simulink model "roverClosed_states_hw"  (R2024a)
settings: Solver=FixedStepAuto  StartTime=0.0  StopTime=100  FixedStep=TS  RelTol=1e-3  EnableMultiTasking=on
PostLoadFcn:
  | params
  | load('motorResponse.mat')
model workspace (MAT data in the model file):
  TS = 0.01
undefined symbols (not defined in the file): L, PWMcmdMono, r, speedMono, StartTheta
libraries: arduinomotorcarrierlib x4, simulink_extras x4, slpidlib x2
settings Model: ExtModeTrigDuration=2  Creator=jmodiset  LastModifiedBy=Sheen
settings SolverCC: AlgebraicLoopSolver=TrustRegion
settings DataIOCC: ReturnWorkspaceOutputs=off
settings OptimizationCC: PassReuseOutputArgsThreshold=0  MaxStackSize=64
settings DebuggingCC: UnderspecifiedInitializationDetection=Classic  MergeDetectMultiDrivingBlocksExec=none  ParameterTunabilityLossMsg=error  UnconnectedInputMsg=warning  UnconnectedOutputMsg=warning  UnconnectedLineMsg=warning  PregeneratedLibrarySubsystemCodeDiagnostic=none  ArithmeticOperatorsInVariantConditions=warning
settings HardwareCC: ProdBitPerPointer=32  ProdBitPerSizeT=32  ProdBitPerPtrDiffT=32  ProdLargestAtomicInteger=Long  ProdLargestAtomicFloat=Double  ProdWordSize=32  ProdHWDeviceType=ARM Compatible->ARM Cortex  UseEmbeddedCoderFeatures=off  UseSimulinkCoderFeatures=off
settings ModelReferenceCC: EnableRefExpFcnMdlSchedulingChecks=on
settings SFSimCC: SimUseLocalCustomCode=off  MATLABDynamicMemAlloc=off  CustomCodeUndefinedFunction=UseInterfaceOnly
settings RTWCC: Description=Embedded Coder  SystemTargetFile=ert.tlc  HardwareBoard=Arduino Nano 33 IoT  TemplateMakefile=ert_default_tmf  RTWUseLocalCustomCode=off  Toolchain=Arduino ARM  BuildConfiguration=Faster Runs  GPUComputeCapability=3.5
settings CodeAppCC: ForceParamTrailComments=on  OperatorAnnotations=on
settings ERTTargetCC: ERTCustomFileBanners=off  SupportContinuousTime=on  SupportNonInlinedSFcns=on  RemoveResetFunc=off  SupportVariableSizeSignals=on  ModelStepFunctionPrototypeControlCompliant=off  ExtModeStaticAllocSize=8192

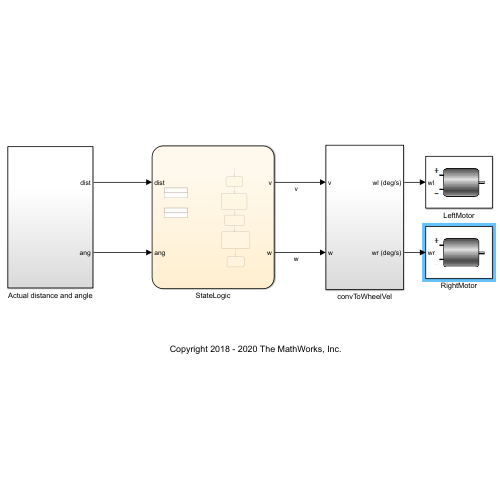
[thumbnail: Simulink's stored preview of the top-level diagram]
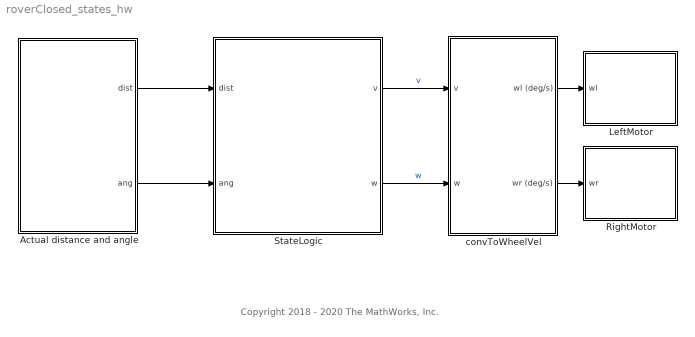
== system roverClosed_states_hw ==
  note: Copyright 2018 - 2020 The MathWorks, Inc.
  Actual distance and angle : Subsystem
  LeftMotor : Subsystem
      mask Display:
      | color('white');
      | plot([100,100,100,100]*1,[100,100,100,100]*1);
      | plot([100,100,100,100]*0,[100,100,100,100]*0);
      | sppkgroot = strrep(codertarget.arduinobase.internal.getBaseSpPkgRootDir(),'\','/');
      | image(fullfile(sppkgroot,'resources','dcmotor.png'),'center')
  RightMotor : Subsystem
      mask Display:
      | color('white');
      | plot([100,100,100,100]*1,[100,100,100,100]*1);
      | plot([100,100,100,100]*0,[100,100,100,100]*0);
      | sppkgroot = strrep(codertarget.arduinobase.internal.getBaseSpPkgRootDir(),'\','/');
      | image(fullfile(sppkgroot,'resources','dcmotor.png'),'center')
  StateLogic : Stateflow chart  TreatAsAtomicUnit=on
  convToWheelVel : Subsystem
  wires:
  Actual distance and angle/1(dist) -> StateLogic/1(dist)
  Actual distance and angle/2(ang) -> StateLogic/2(ang)
  convToWheelVel/1(wl (deg/s)) -> LeftMotor/1(wl)
  StateLogic/1(v) -> convToWheelVel/1(v)  "v"
  convToWheelVel/2(wr (deg/s)) -> RightMotor/1(wr)
  StateLogic/2(w) -> convToWheelVel/2(w)  "w"

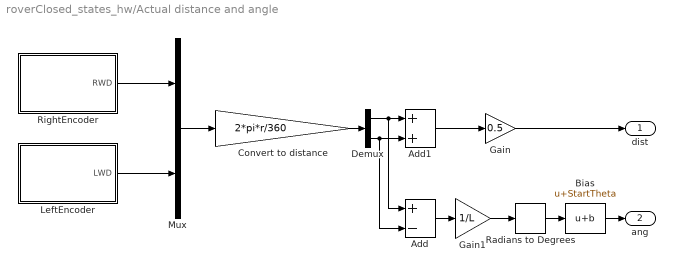
== system roverClosed_states_hw/Actual distance and angle ==
  Add : Sum  Inputs=+-
  Add1 : Sum
  Bias : Bias  Bias=StartTheta  SaturateOnIntegerOverflow=off
  Convert to distance : Gain  Gain=2*pi*r/360
  Demux : Demux  Outputs=2
  Gain : Gain  Gain=0.5
  Gain1 : Gain  Gain=1/L
  LeftEncoder : Subsystem
  Mux : Mux  Inputs=2
  Radians to Degrees : simulink_extras/Transformations/Radians to Degrees
  RightEncoder : Subsystem
  dist : Outport  VectorParamsAs1DForOutWhenUnconnected=off
  ang : Outport  Port=2  VectorParamsAs1DForOutWhenUnconnected=off
  wires:
  RightEncoder/1(RWD) -> Mux/1
  Gain1/1 -> Radians to Degrees/1
  Add/1 -> Gain1/1
  Demux/2 -> Add1/2, Add/2
  Convert to distance/1 -> Demux/1
  Demux/1 -> Add1/1, Add/1
  Mux/1 -> Convert to distance/1
  LeftEncoder/1(LWD) -> Mux/2
  Radians to Degrees/1 -> Bias/1
  Add1/1 -> Gain/1
  Gain/1 -> dist/1
  Bias/1 -> ang/1

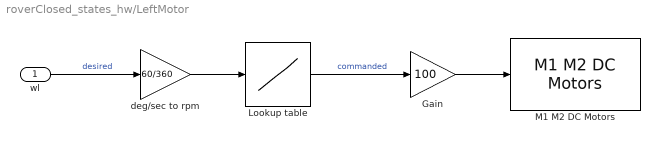
== system roverClosed_states_hw/LeftMotor ==
  wl : Inport
  Gain : Gain  Gain=100
  Lookup table : Lookup_n-D  NumberOfTableDimensions=1  BreakpointsForDimension1=speedMono  Table=PWMcmdMono  UseLastTableValue=on  InternalRulePriority=Speed  RndMeth=Simplest
  M1 M2 DC Motors : arduinomotorcarrierlib/M1 M2 DC Motors  SlaveAddress=uint8( hex2dec( '66' ) )  blockPlatform=ARDUINO  MotorNumber=M2  MotorCarrierPWMFreq=100
  deg/sec to rpm : Gain  Gain=60/360
  wires:
  wl/1 -> deg/sec to rpm/1  "desired"
  Lookup table/1 -> Gain/1  "commanded"
  deg/sec to rpm/1 -> Lookup table/1
  Gain/1 -> M1 M2 DC Motors/1

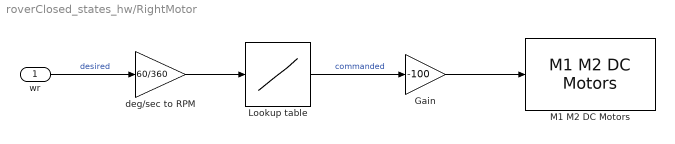
== system roverClosed_states_hw/RightMotor ==
  wr : Inport
  Gain : Gain  Gain=-100
  Lookup table : Lookup_n-D  NumberOfTableDimensions=1  BreakpointsForDimension1=speedMono  Table=PWMcmdMono  UseLastTableValue=on  InternalRulePriority=Speed  RndMeth=Simplest
  M1 M2 DC Motors : arduinomotorcarrierlib/M1 M2 DC Motors  SlaveAddress=uint8( hex2dec( '66' ) )  blockPlatform=ARDUINO  MotorNumber=M1  MotorCarrierPWMFreq=100
  deg/sec to RPM : Gain  Gain=60/360
  wires:
  wr/1 -> deg/sec to RPM/1  "desired"
  Lookup table/1 -> Gain/1  "commanded"
  Gain/1 -> M1 M2 DC Motors/1
  deg/sec to RPM/1 -> Lookup table/1

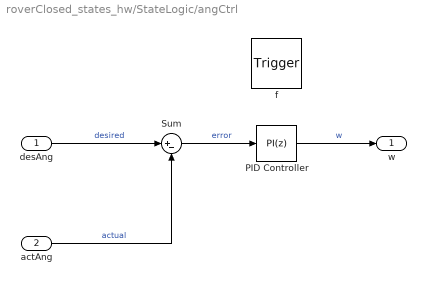
== system roverClosed_states_hw/StateLogic/angCtrl ==
  desAng : Inport  OutDataTypeStr=double  PortDimensions=1
  actAng : Inport  Port=2  OutDataTypeStr=double  PortDimensions=1
  f : TriggerPort  TriggerType=function-call  VariantControl=(inherit)
      settings: CopyFcn=Stateflow.SLINSF.SimulinkMan.removeBlockPreDeleteFcn  PreDeleteFcn=Stateflow.SLINSF.SimulinkMan.unsafePredeleteFcn
  PID Controller : slpidlib/PID Controller  Controller=PI  Form=Parallel  TimeDomain=Discrete-time  UseExternalTs=off  SampleTime=-1  IntegratorMethod=Forward Euler  FilterMethod=Forward Euler  ControllerParametersSource=internal  P=2  I=0.2  UseKiTs=off  D=0  UseExternalDerivativeSource=off  N=100  UseFilter=on  TunerSelectOption=Transfer Function Based (PID Tuner App)  InitialConditionSource=internal  InitialConditionForIntegrator=0  InitialConditionForFilter=0  DifferentiatorICPrevScaledInput=0  ExternalReset=none  TrackingMode=off  Kt=1  LimitOutput=off  SatLimitsSource=internal  UpperSaturationLimit=inf  LowerSaturationLimit=-inf  LinearizeAsGain=on  AntiWindupMode=none  Kb=1  LimitIntegrator=off  UpperIntegratorSaturationLimit=inf  LowerIntegratorSaturationLimit=-inf  POutMin=[]  POutMax=[]  IOutMin=[]  IOutMax=[]  DOutMin=[]  DOutMax=[]  NOutMin=[]  NOutMax=[]  SumOutMin=[]  SumOutMax=[]  SaturationOutMin=[]  SaturationOutMax=[]  PParamMin=[]  PParamMax=[]  IParamMin=[]  IParamMax=[]  DParamMin=[]  DParamMax=[]  NParamMin=[]  NParamMax=[]  KbParamMin=[]  KbParamMax=[]  KtParamMin=[]  KtParamMax=[]  KbOutMin=[]  KbOutMax=[]  KtOutMin=[]  KtOutMax=[]  IntegratorOutMin=[]  IntegratorOutMax=[]  FilterOutMin=[]  FilterOutMax=[]  SumI1OutMin=[]  SumI1OutMax=[]  SumI2OutMin=[]  SumI2OutMax=[]  SumI3OutMin=[]  SumI3OutMax=[]  SumI4OutMin=[]  SumI4OutMax=[]  SumDOutMin=[]  SumDOutMax=[]  DifferentiatorOutMin=[]  DifferentiatorOutMax=[]  FilterDiffOutCoefMin=[]  FilterDiffOutCoefMax=[]  ReciprocalOutMin=[]  ReciprocalOutMax=[]  SumDenOutMin=[]  SumDenOutMax=[]  SumNumOutMin=[]  SumNumOutMax=[]  DivideOutMin=[]  DivideOutMax=[]  UdiffTsProdOutMin=[]  UdiffTsProdOutMax=[]  NTsProdOutMin=[]  NTsProdOutMax=[]  UintegralTsProdOutMin=[]  UintegralTsProdOutMax=[]  UngainTsProdOutMin=[]  UngainTsProdOutMax=[]  ClampingZeroOutDataTypeStr=Inherit: Inherit via back propagation  ClampingZeroOutMin=[]  ClampingZeroOutMax=[]  FilterDenConstantOutDataTypeStr=Inherit: Inherit via back propagation  FilterDenConstantOutMin=[]  FilterDenConstantOutMax=[]  PCopyOutDataTypeStr=Inherit: Inherit via back propagation  PCopyOutMin=[]  PCopyOutMax=[]  NCopyOutDataTypeStr=Inherit: Inherit via back propagation  NCopyOutMin=[]  NCopyOutMax=[]  IntegratorContinuousStateAttributes=''  IntegratorStateMustResolveToSignalObject=off  IntegratorRTWStateStorageClass=Auto  FilterContinuousStateAttributes=''  FilterStateMustResolveToSignalObject=off  FilterRTWStateStorageClass=Auto  ParallelPVariant=InternalParameters  IdealPVariant=Disabled  IVariant=InternalParameters  DVariant=Disabled  IntegratorVariant=Discrete  SatVariant=Disabled  AWVariant=Passthrough  PCopyVariant=Disabled  TRVariant=Disabled  FdbkBlocksVariant=Forward  IdealPFdbkVariant=Disabled  SatFdbkVariant=Disabled  DerivativeFilterVariant=Disabled  NVariant=Disabled  NCopyVariant=Disabled_SignalSpec  FilterICVariant=Disabled  IntegratorICVariant=InternalICs  ExternalResetVariant=Disabled  TRSumVariant=Passthrough  SumFdbkVariant=Disabled  SumVariant=Sum_PI  TsampFilterVariant=InternalTs  TsampNgainVariant=Passthrough  TsampIntegralVariant=Disabled_SignalSpec  ExternalSaturationOutDataTypeStr=Inherit: Same as second input  DerivativeSourceVariant=Disabled
  Sum : Sum  Inputs=|+-
  w : Outport  VectorParamsAs1DForOutWhenUnconnected=off
  wires:
  actAng/1 -> Sum/2  "actual"
  desAng/1 -> Sum/1  "desired"
  PID Controller/1 -> w/1  "w"
  Sum/1 -> PID Controller/1  "error"

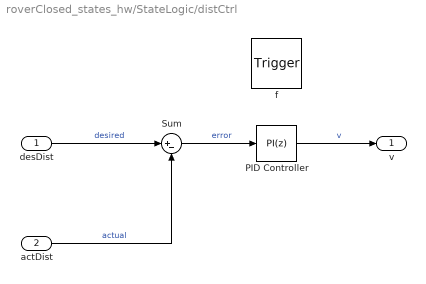
== system roverClosed_states_hw/StateLogic/distCtrl ==
  desDist : Inport  OutDataTypeStr=double  PortDimensions=1
  actDist : Inport  Port=2  OutDataTypeStr=double  PortDimensions=1
  f : TriggerPort  TriggerType=function-call  VariantControl=(inherit)
      settings: CopyFcn=Stateflow.SLINSF.SimulinkMan.removeBlockPreDeleteFcn  PreDeleteFcn=Stateflow.SLINSF.SimulinkMan.unsafePredeleteFcn
  PID Controller : slpidlib/PID Controller  Controller=PI  Form=Parallel  TimeDomain=Discrete-time  UseExternalTs=off  SampleTime=-1  IntegratorMethod=Forward Euler  FilterMethod=Forward Euler  ControllerParametersSource=internal  P=0.2  I=0.001  UseKiTs=off  D=0  UseExternalDerivativeSource=off  N=100  UseFilter=on  TunerSelectOption=Transfer Function Based (PID Tuner App)  InitialConditionSource=internal  InitialConditionForIntegrator=0  InitialConditionForFilter=0  DifferentiatorICPrevScaledInput=0  ExternalReset=none  TrackingMode=off  Kt=1  LimitOutput=off  SatLimitsSource=internal  UpperSaturationLimit=inf  LowerSaturationLimit=-inf  LinearizeAsGain=on  AntiWindupMode=none  Kb=1  LimitIntegrator=off  UpperIntegratorSaturationLimit=inf  LowerIntegratorSaturationLimit=-inf  POutMin=[]  POutMax=[]  IOutMin=[]  IOutMax=[]  DOutMin=[]  DOutMax=[]  NOutMin=[]  NOutMax=[]  SumOutMin=[]  SumOutMax=[]  SaturationOutMin=[]  SaturationOutMax=[]  PParamMin=[]  PParamMax=[]  IParamMin=[]  IParamMax=[]  DParamMin=[]  DParamMax=[]  NParamMin=[]  NParamMax=[]  KbParamMin=[]  KbParamMax=[]  KtParamMin=[]  KtParamMax=[]  KbOutMin=[]  KbOutMax=[]  KtOutMin=[]  KtOutMax=[]  IntegratorOutMin=[]  IntegratorOutMax=[]  FilterOutMin=[]  FilterOutMax=[]  SumI1OutMin=[]  SumI1OutMax=[]  SumI2OutMin=[]  SumI2OutMax=[]  SumI3OutMin=[]  SumI3OutMax=[]  SumI4OutMin=[]  SumI4OutMax=[]  SumDOutMin=[]  SumDOutMax=[]  DifferentiatorOutMin=[]  DifferentiatorOutMax=[]  FilterDiffOutCoefMin=[]  FilterDiffOutCoefMax=[]  ReciprocalOutMin=[]  ReciprocalOutMax=[]  SumDenOutMin=[]  SumDenOutMax=[]  SumNumOutMin=[]  SumNumOutMax=[]  DivideOutMin=[]  DivideOutMax=[]  UdiffTsProdOutMin=[]  UdiffTsProdOutMax=[]  NTsProdOutMin=[]  NTsProdOutMax=[]  UintegralTsProdOutMin=[]  UintegralTsProdOutMax=[]  UngainTsProdOutMin=[]  UngainTsProdOutMax=[]  ClampingZeroOutDataTypeStr=Inherit: Inherit via back propagation  ClampingZeroOutMin=[]  ClampingZeroOutMax=[]  FilterDenConstantOutDataTypeStr=Inherit: Inherit via back propagation  FilterDenConstantOutMin=[]  FilterDenConstantOutMax=[]  PCopyOutDataTypeStr=Inherit: Inherit via back propagation  PCopyOutMin=[]  PCopyOutMax=[]  NCopyOutDataTypeStr=Inherit: Inherit via back propagation  NCopyOutMin=[]  NCopyOutMax=[]  IntegratorContinuousStateAttributes=''  IntegratorStateMustResolveToSignalObject=off  IntegratorRTWStateStorageClass=Auto  FilterContinuousStateAttributes=''  FilterStateMustResolveToSignalObject=off  FilterRTWStateStorageClass=Auto  ParallelPVariant=InternalParameters  IdealPVariant=Disabled  IVariant=InternalParameters  DVariant=Disabled  IntegratorVariant=Discrete  SatVariant=Disabled  AWVariant=Passthrough  PCopyVariant=Disabled  TRVariant=Disabled  FdbkBlocksVariant=Forward  IdealPFdbkVariant=Disabled  SatFdbkVariant=Disabled  DerivativeFilterVariant=Disabled  NVariant=Disabled  NCopyVariant=Disabled_SignalSpec  FilterICVariant=Disabled  IntegratorICVariant=InternalICs  ExternalResetVariant=Disabled  TRSumVariant=Passthrough  SumFdbkVariant=Disabled  SumVariant=Sum_PI  TsampFilterVariant=InternalTs  TsampNgainVariant=Passthrough  TsampIntegralVariant=Disabled_SignalSpec  ExternalSaturationOutDataTypeStr=Inherit: Same as second input  DerivativeSourceVariant=Disabled
  Sum : Sum  Inputs=|+-
  v : Outport  VectorParamsAs1DForOutWhenUnconnected=off
  wires:
  actDist/1 -> Sum/2  "actual"
  desDist/1 -> Sum/1  "desired"
  PID Controller/1 -> v/1  "v"
  Sum/1 -> PID Controller/1  "error"

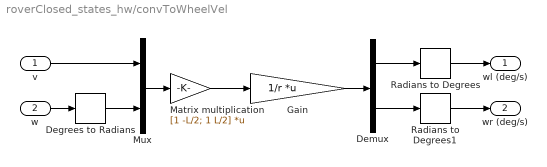
== system roverClosed_states_hw/convToWheelVel ==
  v : Inport
  w : Inport  Port=2
  " Gain" : Gain  Gain=1/r  Multiplication=Matrix(K*u)
  Degrees to Radians : simulink_extras/Transformations/Degrees to Radians
  Demux : Demux  Outputs=2
  Matrix multiplication : Gain  Gain=[1 -L/2; 1 L/2]  Multiplication=Matrix(K*u)
  Mux : Mux  Inputs=2
  Radians to Degrees : simulink_extras/Transformations/Radians to Degrees
  Radians to Degrees1 : simulink_extras/Transformations/Radians to Degrees
  wl (deg/s) : Outport  VectorParamsAs1DForOutWhenUnconnected=off
  wr (deg/s) : Outport  Port=2  VectorParamsAs1DForOutWhenUnconnected=off
  wires:
  " Gain"/1 -> Demux/1
  Matrix multiplication/1 -> " Gain"/1
  v/1 -> Mux/1
  Mux/1 -> Matrix multiplication/1
  Demux/1 -> Radians to Degrees/1
  Demux/2 -> Radians to Degrees1/1
  w/1 -> Degrees to Radians/1
  Radians to Degrees/1 -> wl (deg/s)/1
  Radians to Degrees1/1 -> wr (deg/s)/1
  Degrees to Radians/1 -> Mux/2

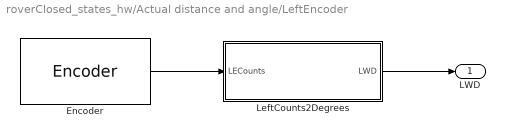
== system roverClosed_states_hw/Actual distance and angle/LeftEncoder ==
  Encoder : arduinomotorcarrierlib/Encoder  SlaveAddress=uint8( hex2dec( '66' ) )  blockPlatform=ARDUINO  Encoder=2  ShowSpeed=off  ResetOption=on  SampleTime=0.01
  LeftCounts2Degrees : Subsystem
  LWD : Outport  VectorParamsAs1DForOutWhenUnconnected=off
  wires:
  LeftCounts2Degrees/1(LWD) -> LWD/1
  Encoder/1 -> LeftCounts2Degrees/1(LECounts)

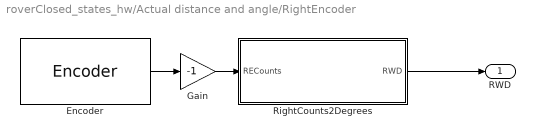
== system roverClosed_states_hw/Actual distance and angle/RightEncoder ==
  Encoder : arduinomotorcarrierlib/Encoder  SlaveAddress=uint8( hex2dec( '66' ) )  blockPlatform=ARDUINO  Encoder=1  ShowSpeed=off  ResetOption=on  SampleTime=0.01
  Gain : Gain  Gain=-1
  RightCounts2Degrees : Subsystem
  RWD : Outport  VectorParamsAs1DForOutWhenUnconnected=off
  wires:
  RightCounts2Degrees/1(RWD) -> RWD/1
  Encoder/1 -> Gain/1
  Gain/1 -> RightCounts2Degrees/1(RECounts)

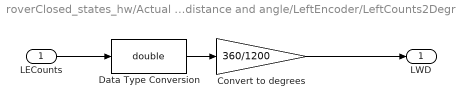
== system roverClosed_states_hw/Actual distance and angle/LeftEncoder/LeftCounts2Degrees ==
  LECounts : Inport
  Convert to degrees : Gain  Gain=360/1200
  Data Type Conversion : DataTypeConversion  OutDataTypeStr=double  SaturateOnIntegerOverflow=off  RndMeth=Floor
  LWD : Outport  VectorParamsAs1DForOutWhenUnconnected=off
  wires:
  LECounts/1 -> Data Type Conversion/1
  Data Type Conversion/1 -> Convert to degrees/1
  Convert to degrees/1 -> LWD/1

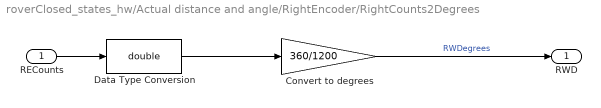
== system roverClosed_states_hw/Actual distance and angle/RightEncoder/RightCounts2Degrees ==
  RECounts : Inport
  Convert to degrees : Gain  Gain=360/1200
  Data Type Conversion : DataTypeConversion  OutDataTypeStr=double  SaturateOnIntegerOverflow=off  RndMeth=Floor
  RWD : Outport  VectorParamsAs1DForOutWhenUnconnected=off
  wires:
  Data Type Conversion/1 -> Convert to degrees/1
  RECounts/1 -> Data Type Conversion/1
  Convert to degrees/1 -> RWD/1  "RWDegrees"

== stateflow chart roverClosed_states_hw/StateLogic ==
  state StopFirst
    entry:
    v = 0; w= 0;
  state v = distCtrl(desDist,actDist) [function]
  state MoveForward
    entry:
    desDist = 30;
    during, exit:
    v = distCtrl(desDist,dist);
    w = 0;
  state w = angCtrl(desAng,actAng) [function]
  state Pause
    entry:
    v = 0;
    w = 0;
  state Turn
    entry:
    desAng = 180;
    during, exit:
    v = 0;
    w = angCtrl(desAng,ang);
  state Stop
    entry:
    v = 0;
    w = 0;
  (default) -> StopFirst
  StopFirst -> MoveForward : after(1,sec)
  MoveForward -> Pause : [abs(desDist - dist) < 0.5]
  Pause -> Turn : after(1,sec)
  Turn -> Stop : [abs(desAng - ang) < 2]
  data: desDist function_input double size=1; actDist function_input double size=1; v function_output; desAng function_input double size=1; actAng function_input double size=1; w function_output; dist input; ang input; v output; w output; desDist local; desAng local
